simulink model "Electromech_sys_deformation_lin_obs"  (R2025b)
settings: Solver=VariableStepAuto  StartTime=0.0  StopTime=10.0  RelTol=1e-3
values from neighbouring files (symbols this model uses):
  A = (J - R) * Hxx    [linearize_electromech.m]    (also in linearize_mech.m = (J - R) * Hxx + grad_g * u_eq_mech)
  B = g    [linearize_electromech.m]    (also in linearize_mech.m)
  p_0 = 0    [Init_Simulink_param_lin_Electromech.m]
  ptilde_0 = phat_0 - x_eq(2)    [Init_Simulink_param_lin_Electromech.m]
  q_0 = 0    [Init_Simulink_param_lin_Electromech.m]
  Q_0 = 0    [Init_Simulink_param_lin_Electromech.m]
  qtilde_0 = qhat_0 - x_eq(1)    [Init_Simulink_param_lin_Electromech.m]
  Qtilde_0 = Qhat_0 - x_eq(3)    [Init_Simulink_param_lin_Electromech.m]
  x_eq = [q_eq; p_eq; Q_eq]    [equilibrium_electromech.m]
undefined symbols (not defined in the file or in its folder): params, u_eq
settings Model: Creator=filippougolini  LastModifiedBy=filippougolini

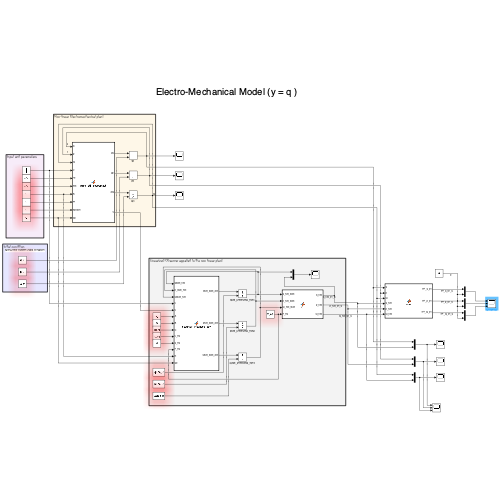
[thumbnail: Simulink's stored preview of the top-level diagram]
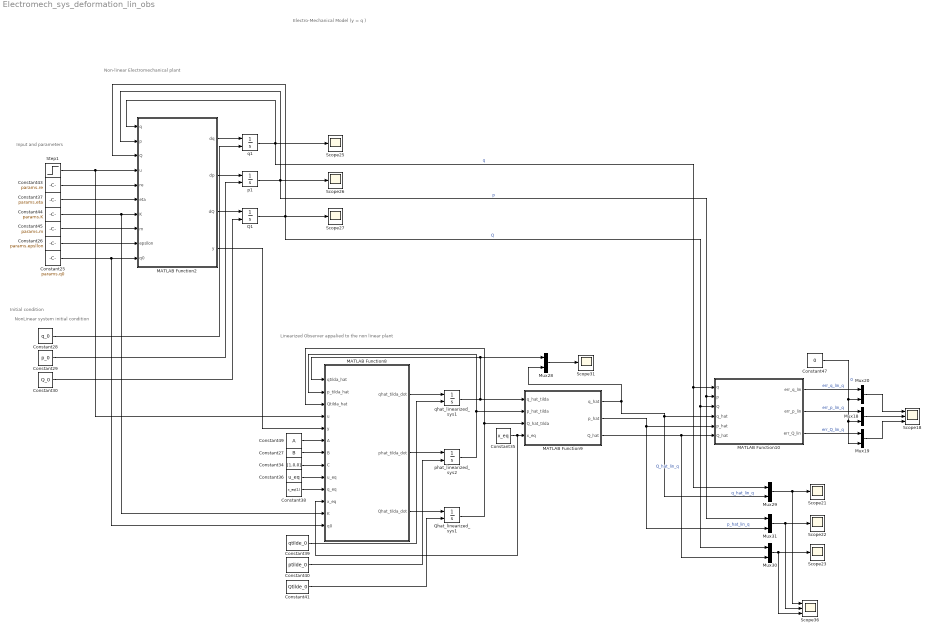
== system Electromech_sys_deformation_lin_obs ==
  note: Input and parameters
  note: Linearized Observer appalied to the non linear plant
  note: NonLinear system initial condition
  note: Non-linear Electromechanical plant
  note: Electro-Mechanical Model (y = q )
  note: Initial condition
  Constant25 : Constant  Value=params.q0
  Constant26 : Constant  Value=params.epsllon
  Constant27 : Constant  Value=B
  Constant28 : Constant  Value=q_0
  Constant29 : Constant  Value=p_0
  Constant30 : Constant  Value=Q_0
  Constant34 : Constant  Value=[1,0,0]
  Constant35 : Constant  Value=x_eq
  Constant36 : Constant  Value=u_eq
  Constant37 : Constant  Value=params.eta
  Constant38 : Constant  Value=x_eq(1)
  Constant39 : Constant  Value=qtilde_0
  Constant40 : Constant  Value=ptilde_0
  Constant41 : Constant  Value=Qtilde_0
  Constant43 : Constant  Value=params.re
  Constant44 : Constant  Value=params.K
  Constant45 : Constant  Value=params.m
  Constant47 : Constant  Value=0
  Constant49 : Constant  Value=A
  MATLAB Function10 : MATLAB Function  TreatAsAtomicUnit=on
  MATLAB Function2 : MATLAB Function  TreatAsAtomicUnit=on
  MATLAB Function8 : MATLAB Function  TreatAsAtomicUnit=on
  MATLAB Function9 : MATLAB Function  TreatAsAtomicUnit=on
  Mux{18..20,28..31} (7 alike) : Mux  Inputs=2
  Q1 : Integrator  InitialConditionSource=external
  Qhat_linearized_sys1 : Integrator  InitialConditionSource=external  InitialCondition=20e-5
  Scope18 : Scope  NumInputPorts=3
      settings: ActiveDisplayYMinimum=-0.010993446298248871  ActiveDisplayYMaximum=0.012696753596182685  DataLoggingVariableName=ScopeData18
  Scope{21..23,25..27,31} (7 alike) : Scope
      Scope21 settings: ActiveDisplayYMinimum=-0.00014562196235781276  ActiveDisplayYMaximum=0.0013105976612203152  DataLoggingVariableName=ScopeData21
      Scope22 settings: ActiveDisplayYMinimum=-0.0045902088543352884  ActiveDisplayYMaximum=0.00516486271210546  DataLoggingVariableName=ScopeData22
      Scope23 settings: ActiveDisplayYMinimum=-2.096197823231283E-8  ActiveDisplayYMaximum=1.8865780409081551E-7  DataLoggingVariableName=ScopeData23
      Scope25 settings: ActiveDisplayYMinimum=-4.0944874698701246E-5  ActiveDisplayYMaximum=0.0003685038722883113  DataLoggingVariableName=ScopeData25
      Scope26 settings: ActiveDisplayYMinimum=-1  ActiveDisplayYMaximum=1  DataLoggingVariableName=ScopeData26
      Scope27 settings: ActiveDisplayYMinimum=-1  ActiveDisplayYMaximum=1  DataLoggingVariableName=ScopeData27
      Scope31 settings: ActiveDisplayYMinimum=-0.0028704641819507128  ActiveDisplayYMaximum=0.00068289488649407159  DataLoggingVariableName=ScopeData31
  Scope36 : Scope  NumInputPorts=3
      settings: ActiveDisplayString=3  ActiveDisplayYMinimum=-3.7694718700971209E-7  ActiveDisplayYMaximum=9.7438576334412446E-8  DataLoggingVariableName=ScopeData36
  Step1 : Step  After=5e3  SampleTime=0
  p1 : Integrator  InitialConditionSource=external
  phat_linearized_sys2 : Integrator  InitialConditionSource=external  InitialCondition=20e-5
  q1 : Integrator  InitialConditionSource=external
  qhat_linearized_sys1 : Integrator  InitialConditionSource=external  InitialCondition=20e-5
  wires:
  Mux18/1 -> Scope18/2
  Mux28/1 -> Scope31/1
  Constant36/1 -> MATLAB Function8/9(u_eq)
  Mux19/1 -> Scope18/3
  MATLAB Function10/3(err_Q_lin) -> Mux19/1  "err_Q_lin_q"
  Constant49/1 -> MATLAB Function8/6(A)
  Constant39/1 -> qhat_linearized_sys1/2
  Step1/1 -> MATLAB Function2/4(u), MATLAB Function8/4(u)
  Constant29/1 -> p1/2
  MATLAB Function2/2(dp) -> p1/1
  MATLAB Function9/3(Q_hat) -> MATLAB Function10/6(Q_hat), Mux30/2  "Q_hat_lin_q"
  MATLAB Function8/3(Qhat_tilda_dot) -> Qhat_linearized_sys1/1
  MATLAB Function2/1(dq) -> q1/1
  MATLAB Function8/1(qhat_tilda_dot) -> qhat_linearized_sys1/1
  MATLAB Function8/2(phat_tilda_dot) -> phat_linearized_sys2/1
  MATLAB Function2/3(dQ) -> Q1/1
  Constant28/1 -> q1/2
  Constant44/1 -> MATLAB Function2/7(K), MATLAB Function8/12(K)
  MATLAB Function10/2(err_p_lin) -> Mux18/1  "err_p_lin_q"
  Qhat_linearized_sys1/1 -> MATLAB Function8/3(Qtilda_hat), MATLAB Function9/3(Q_hat_tilda)
  p1/1 -> Mux31/1, MATLAB Function10/2(p), Scope26/1, MATLAB Function2/2(p)  "p"
  Constant27/1 -> MATLAB Function8/7(B)
  Constant26/1 -> MATLAB Function2/9(epsllon)
  Mux31/1 -> Scope36/2, Scope22/1
  Constant35/1 -> MATLAB Function8/11(x_eq), MATLAB Function9/4(x_eq)
  Constant30/1 -> Q1/2
  MATLAB Function10/1(err_q_lin) -> Mux20/1  "err_q_lin_q"
  Constant38/1 -> MATLAB Function8/10(q_eq)
  Mux29/1 -> Scope36/1, Scope21/1
  Constant47/1 -> Mux19/2, Mux18/2, Mux20/2  "0"
  Constant37/1 -> MATLAB Function2/6(eta)
  Constant34/1 -> MATLAB Function8/8(C)
  Mux20/1 -> Scope18/1
  MATLAB Function2/4(y) -> MATLAB Function8/5(y)
  Q1/1 -> MATLAB Function10/3(Q), Mux30/1, Scope27/1, MATLAB Function2/3(Q)  "Q"
  Constant41/1 -> Qhat_linearized_sys1/2
  qhat_linearized_sys1/1 -> MATLAB Function8/1(qtilda_hat), Mux28/1, MATLAB Function9/1(q_hat_tilda)
  Mux30/1 -> Scope36/3, Scope23/1
  Constant43/1 -> MATLAB Function2/5(re)
  phat_linearized_sys2/1 -> MATLAB Function8/2(p_tilda_hat), MATLAB Function9/2(p_hat_tilda)
  Constant45/1 -> MATLAB Function2/8(m)
  MATLAB Function9/2(p_hat) -> Mux31/2, MATLAB Function10/5(p_hat)  "p_hat_lin_q"
  q1/1 -> MATLAB Function2/1(q), Scope25/1, MATLAB Function10/1(q), Mux29/1  "q"
  Constant25/1 -> MATLAB Function2/10(q0), MATLAB Function8/13(q0)
  MATLAB Function9/1(q_hat) -> Mux28/2, Mux29/2, MATLAB Function10/4(q_hat)  "q_hat_lin_q"
  Constant40/1 -> phat_linearized_sys2/2

== matlab function Electromech_sys_deformation_lin_obs/MATLAB Function8 ==
  data: qhat_tilda_dot output; phat_tilda_dot output; Qhat_tilda_dot output; qtilda_hat input; p_tilda_hat input; Qtilda_hat input; u input; y input; A input; B input; C input; u_eq input; q_eq input; x_eq input; K input; q0 input
function [qhat_tilda_dot, phat_tilda_dot, Qhat_tilda_dot] = ...
    observer_linearized_dev(qtilda_hat, p_tilda_hat, Qtilda_hat, u, y, A, ...
    B, C, u_eq, q_eq, x_eq, K, q0)

    % ---- Deviation state and absolute estimate ---- 
    delta_xhat = [qtilda_hat; p_tilda_hat; Qtilda_hat]; % 3x1 
    % ---- Deviation input and output ---- 
    delta_u = u - u_eq; 
    delta_y = y - q_eq;
    Qhat = x_eq(3) + Qtilda_hat;
    qhat = x_eq(1) + qtilda_hat;

    psi_hat = [1/K ; 0; 2*Qhat/(K * (qhat + q0))];

    alpha = 100;
    Lcol = alpha * psi_hat;

    delta_xhatdot = A*delta_xhat + B*delta_u + Lcol* (delta_y - C'*delta_xhat);
    

    % ---- Derivatives of deviation states ---- 
    qhat_tilda_dot = delta_xhatdot(1); 
    phat_tilda_dot = delta_xhatdot(2); 
    Qhat_tilda_dot = delta_xhatdot(3);
end

== matlab function Electromech_sys_deformation_lin_obs/MATLAB Function9 ==
  data: q_hat_tilda input; p_hat_tilda input; Q_hat_tilda input; x_eq input; q_hat output; p_hat output; Q_hat output
function [q_hat, p_hat, Q_hat] = fcn(q_hat_tilda, p_hat_tilda, Q_hat_tilda, ...
    x_eq)
    
    q_tilda_eq = x_eq(1);
    p_tilda_eq = x_eq(2);
    Q_tilda_eq = x_eq(3);

    
    
    q_hat = q_hat_tilda + q_tilda_eq;
    p_hat = p_hat_tilda + p_tilda_eq;
    Q_hat = Q_hat_tilda + Q_tilda_eq;
end

== matlab function Electromech_sys_deformation_lin_obs/MATLAB Function10 ==
  data: q input; err_q_lin output; p input; Q input; q_hat input; p_hat input; Q_hat input; err_p_lin output; err_Q_lin output
function [err_q_lin, err_p_lin, err_Q_lin] = error(q, p, Q, q_hat, p_hat, Q_hat)

    err_q_lin = q - q_hat;
    err_p_lin = p - p_hat;
    err_Q_lin = Q - Q_hat;
end

== matlab function Electromech_sys_deformation_lin_obs/MATLAB Function2 ==
  data: q input; p input; Q input; u input; dq output; re input; eta input; K input; m input; epsllon input; q0 input; dp output; dQ output; y output
function [dq, dp, dQ, y] = plant_pH_electromech(q, p, Q, u, re, eta, K, m, epsllon, q0)
% Electro-mechanical pH plant

    % Parameters: m, K, eta, eps, re, q0 in workspace

    J = [  0  1  0;
          -1  0  0;
           0  0  0 ];

    R = diag([0, eta, 1/re]);
    g = [0; 0; 1/re];

    % Hamiltonian gradient gradH(q,p,Q)
    Cq   = epsllon * (q + q0)^4;

    dHdq = K*q - 2*Q^2 / (epsllon * (q + q0)^5);
    dHdp = p / m;
    dHdQ = Q / Cq;

    gradH = [dHdq; dHdp; dHdQ];

    xdot = (J - R) * gradH + g*u;

    y = q; % output is the deformation
    
    dq = xdot(1);
    dp = xdot(2);
    dQ = xdot(3);
end
